simulink model "MultiportSwitch_TestGen15"  (R2017b)
settings: Solver=FixedStepDiscrete  StartTime=0.0  StopTime=10.0  RelTol=1e-3
settings Model: Creator=ktrinh  LastModifiedBy=ktrinh
settings DebuggingCC: ParameterOverflowMsg=none

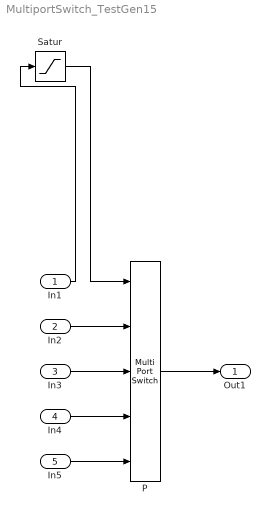
== system MultiportSwitch_TestGen15 ==
  In1 : Inport  OutMin=1  OutMax=4
  In2 : Inport  Port=2  PortDimensions=[2,3]
  In3 : Inport  Port=3  PortDimensions=[2,3]
  In4 : Inport  Port=4  PortDimensions=[2,3]
  In5 : Inport  Port=5  PortDimensions=[2,3]
  P : MultiPortSwitch  DataPortForDefault=Additional data port
  Satur : Saturate  UpperLimit=4  LowerLimit=1
  Out1 : Outport
  wires:
  In2/1 -> P/2
  In3/1 -> P/3
  In4/1 -> P/4
  In5/1 -> P/5
  P/1 -> Out1/1
  In1/1 -> Satur/1
  Satur/1 -> P/1
